simulink model "Junctions3"  (Simulink 5.0)
settings: Solver=ode45  StartTime=0.0  StopTime=10.0  RelTol=1e-3
settings Model: Creator=scaife  LastModifiedBy=scaife  ExtModeAutoUpdateStatusClock=off

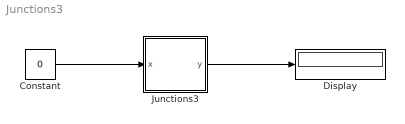
== system Junctions3 ==
  Constant : Constant  Value=0
  Display : Display
  Junctions3 : Stateflow chart
  wires:
  Constant/1 -> Junctions3/1(x)
  Junctions3/1(y) -> Display/1

== stateflow chart Junctions3 ==
  state A
  state B
  (default) -> A
  A -> (junction 5) : [x==0]{y=0}
  (junction 5) -> (junction 6) : [y==0]{y++}
  (junction 6) -> (junction 7) : [y==1]{y++}
  (junction 7) -> (junction 8) : [y==2]{y++}
  (junction 8) -> B : {y++}
  data: x input int32; y output int32 =111111
